simulink model "task_4_reg_obs"  (R2021b)
settings: Solver=FixedStepAuto  StartTime=0.0  StopTime=6.5  FixedStep=0.00005  RelTol=1e-3
settings Model: Creator=den  LastModifiedBy=den

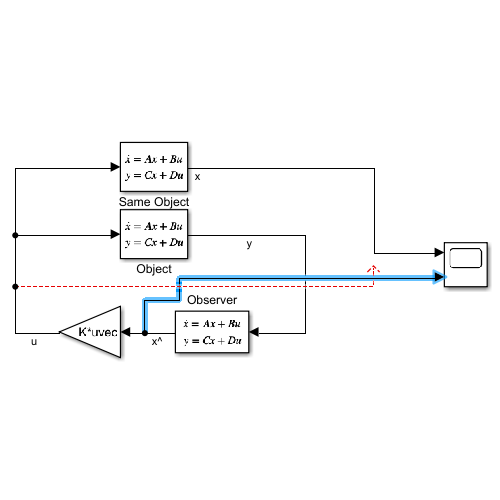
[thumbnail: Simulink's stored preview of the top-level diagram]
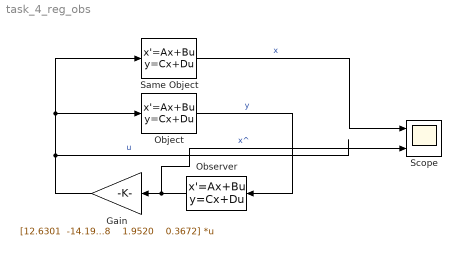
== system task_4_reg_obs ==
  Gain : Gain  Gain="[12.6301  -14.1968    1.9520    0.3672]"  Multiplication=Matrix(K*u) (u vector)
  Object : StateSpace  A=[5 -7 -5 1; -7 5 -1 5; -5 -1 5 7; 1 5 7 5]  B=[5; 7; 1; 9]  C=[0 0 2 2; 1 1 -1 1]  D=[0;0]  InitialCondition=[-3; 17; 2; -8]
  Observer : StateSpace  A="[ 66.1622  -79.9724   84.0899   78.1894;  79.4224  -96.3661  -62.6892  -71.7594;  9.6184  -13.2086  -12.6906   -8.2989; 112.6826 -124.7597    8.9021  -11.3377]"  B="[-38.6708    1.9883; 38.6708    1.9883;8.8272   -1.9883;8.8272    1.9883]"  C=[1 0 0 0; 0 1 0 0; 0 0 1 0; 0 0 0 1]  D=[0 0;0 0;0 0;0 0]  InitialCondition=[5; -1; -8; 12]
  Same Object : StateSpace  A=[5 -7 -5 1; -7 5 -1 5; -5 -1 5 7; 1 5 7 5]  B=[5; 7; 1; 9]  C=[1 0 0 0; 0 1 0 0; 0 0 1 0; 0 0 0 1]  D=[0;0;0;0]  InitialCondition=[-3; 17; 2; -8]
  Scope : Scope  NumInputPorts=2
  wires:
  Object/1 -> Observer/1  "y"
  Observer/1 -> Scope/2, Gain/1  "x^"
  Gain/1 -> Same Object/1, Object/1  "u"
  Same Object/1 -> Scope/1  "x"
